simulink model "lab6_putere"  (R2023b)
settings: Solver=VariableStepAuto  StartTime=0.0  StopTime=10.0  RelTol=1e-3
settings Model: Creator=Daniela  LastModifiedBy=Daniela

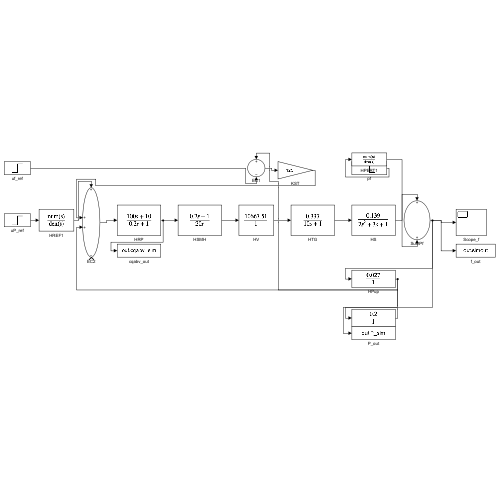
[thumbnail: Simulink's stored preview of the top-level diagram]
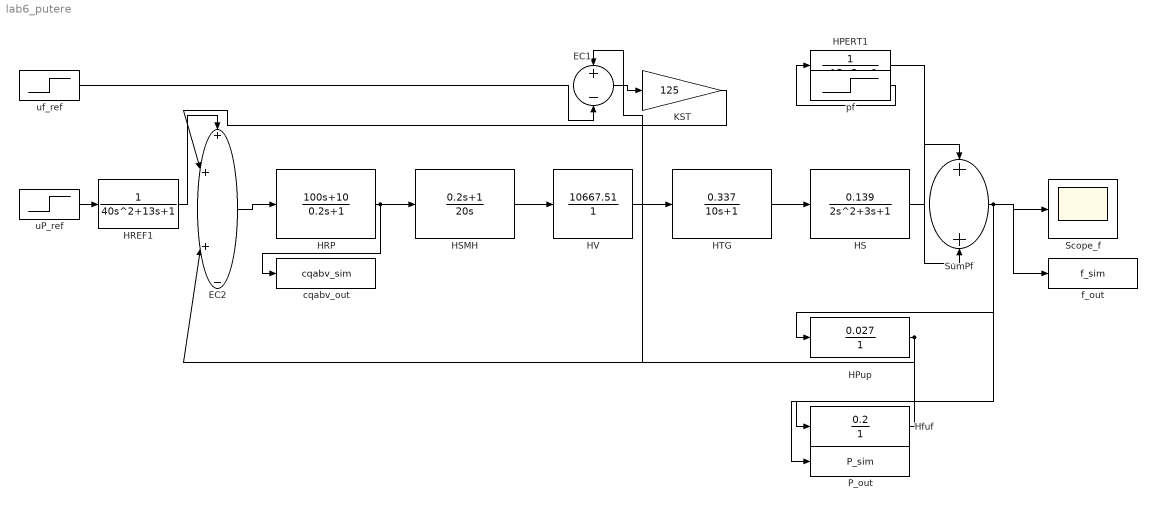
== system lab6_putere ==
  EC1 : Sum  Inputs=+-
  EC2 : Sum  Inputs=+++-
  HPERT1 : TransferFcn  Numerator=1
  HPup : TransferFcn  Numerator=0.027  Denominator=1
  HREF1 : TransferFcn  Numerator=1  Denominator=[40 13 1]
  HRP : TransferFcn  Numerator=[100 10]  Denominator=[0.2 1]
  HS : TransferFcn  Numerator=0.139  Denominator=[2 3 1]
  HSMH : TransferFcn  Numerator=[0.2 1]  Denominator=[20 0]
  HTG : TransferFcn  Numerator=0.337  Denominator=[10 1]
  HV : TransferFcn  Numerator=10667.51  Denominator=1
  Hfuf : TransferFcn  Numerator=0.2  Denominator=1
  KST : Gain  Gain=125
  P_out : ToWorkspace  VariableName=P_sim  SampleTime=-1
  Scope_f : Scope
  SumPf : Sum
  cqabv_out : ToWorkspace  VariableName=cqabv_sim  SampleTime=-1
  f_out : ToWorkspace  VariableName=f_sim  SampleTime=-1
  pf : Step  Time=150  After=-5  SampleTime=0
  uP_ref : Step  Time=0  After=10  SampleTime=0
  uf_ref : Step  Time=0  After=10  SampleTime=0
  wires:
  uP_ref/1 -> HREF1/1
  HREF1/1 -> EC2/1
  EC2/1 -> HRP/1
  HRP/1 -> HSMH/1, cqabv_out/1
  HSMH/1 -> HV/1
  HV/1 -> HTG/1
  HTG/1 -> HS/1
  HS/1 -> SumPf/1
  HPERT1/1 -> SumPf/2
  pf/1 -> HPERT1/1
  SumPf/1 -> Scope_f/1, f_out/1, HPup/1, Hfuf/1
  HPup/1 -> EC2/3, P_out/1
  Hfuf/1 -> EC1/1
  uf_ref/1 -> EC1/2
  EC1/1 -> KST/1
  KST/1 -> EC2/2
